simulink model "ACC_Main"  (R2026a)
settings: Solver=VariableStepAuto  StopTime=30
settings Model: Creator=Quang Huy  LastModifiedBy=ASUS

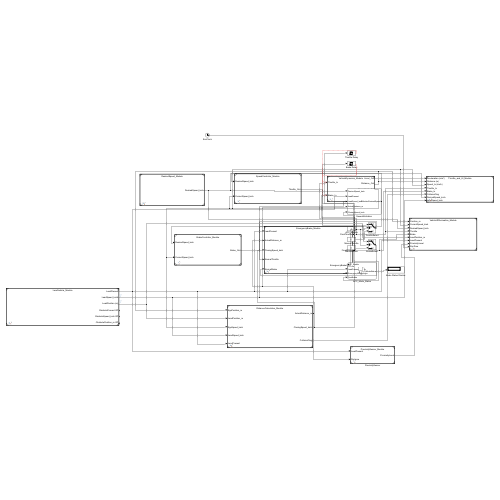
[thumbnail: Simulink's stored preview of the top-level diagram]
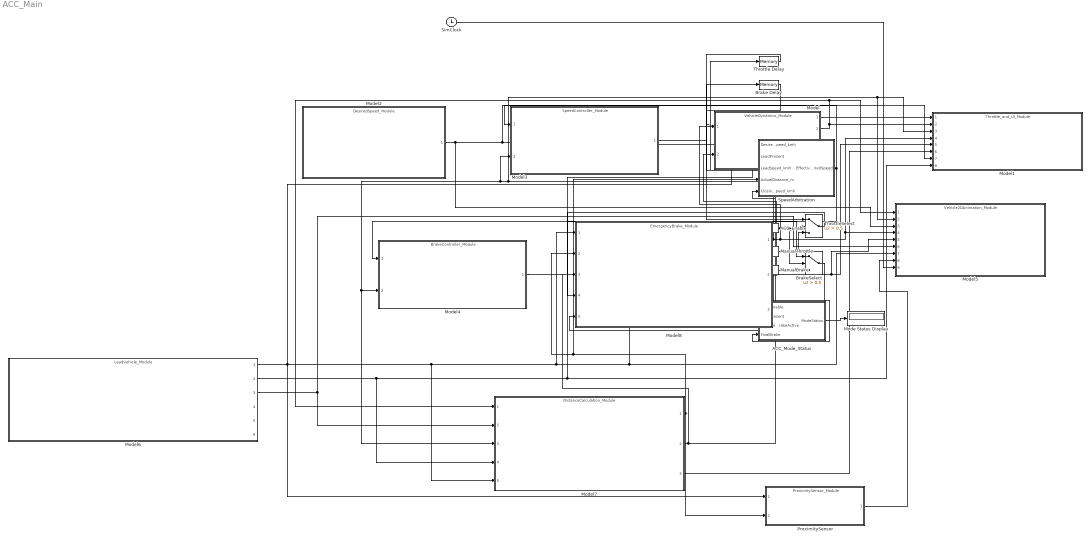
== system ACC_Main ==
  ACC_Enable : Constant  OutDataTypeStr=boolean
  ACC_Mode_Status : Stateflow chart  TreatAsAtomicUnit=on
  Brake Delay : Memory
  BrakeSelect : Switch  Criteria=u2 > Threshold  Threshold=0.5  SaturateOnIntegerOverflow=off  InputSameDT=off
  ManualBrake : Constant  Value=0
  ManualThrottle : Constant  Value=0  OutDataTypeStr=double
  Mode Status Display : Display
  Model : ModelReference  ModelNameDialog=VehicleDynamics_Module.slx  SimulationMode=Normal  ModelReferenceVersion=1.0
  Model1 : ModelReference  ModelNameDialog=Throttle_and_UI_Module.slx  SimulationMode=Normal  ModelReferenceVersion=3.2
  Model2 : ModelReference  ModelNameDialog=DesiredSpeed_Module.slx  SimulationMode=Normal  ModelReferenceVersion=1.0
  Model3 : ModelReference  ModelNameDialog=SpeedController_Module.slx  SimulationMode=Normal  ModelReferenceVersion=1.2
  Model4 : ModelReference  ModelNameDialog=BrakeController_Module.slx  SimulationMode=Normal  ModelReferenceVersion=1.0
  Model5 : ModelReference  ModelNameDialog=Vehicle2DAnimation_Module.slx  SimulationMode=Normal  ModelReferenceVersion=3.1
  Model6 : ModelReference  ModelNameDialog=LeadVehicle_Module.slx  SimulationMode=Normal  ModelReferenceVersion=3.1
  Model7 : ModelReference  ModelNameDialog=DistanceCalculation_Module.slx  SimulationMode=Normal  ModelReferenceVersion=1.0
  Model8 : ModelReference  ModelNameDialog=EmergencyBrake_Module.slx  SimulationMode=Normal  ModelReferenceVersion=1.0
  ProximitySensor : ModelReference  ModelNameDialog=ProximitySensor_Module.slx  SimulationMode=Normal  ModelReferenceVersion=1.2
  SimClock : Clock
  SpeedArbitration : Subsystem
  Throttle Delay : Memory
  ThrottleSelect : Switch  Criteria=u2 > Threshold  Threshold=0.5  SaturateOnIntegerOverflow=off  InputSameDT=off
  wires:
  Model2/1 -> SpeedArbitration/1(DesiredSpeed_kmh), Model1/7, Model5/3
  Model6/3 -> Model7/2, Model5/6
  Model6/2 -> SpeedArbitration/3(LeadSpeed_kmh), Model1/8, Model7/4
  Model8/1 -> Model1/4, Model5/4, Model/1, Throttle Delay/1
  Model8/2 -> Model1/5, Model5/5, Model/2, Brake Delay/1, ACC_Mode_Status/4(FinalBrake)
  Model7/2 -> Model8/3, SpeedArbitration/5(ClosingSpeed_kmh)
  Throttle Delay/1 -> ?
  Brake Delay/1 -> ?
  Model7/3 -> Model1/6
  SpeedArbitration/1(EffectiveDesiredSpeed) -> Model3/1, Model4/1
  Model3/1 -> ThrottleSelect/1
  ACC_Enable/1 -> ThrottleSelect/2, BrakeSelect/2, ACC_Mode_Status/1(ACC_Enable)
  ManualThrottle/1 -> ThrottleSelect/3
  ThrottleSelect/1 -> Model8/4
  Model4/1 -> BrakeSelect/1
  ManualBrake/1 -> BrakeSelect/3
  BrakeSelect/1 -> Model8/5
  Model8/3 -> ACC_Mode_Status/3(EmergencyBrakeActive)
  ACC_Mode_Status/1(ModeStatus) -> Mode Status Display/1
  Model6/1 -> Model5/7, ACC_Mode_Status/2(LeadPresent), Model8/1, Model7/5, ProximitySensor/1, SpeedArbitration/2(LeadPresent)
  Model7/1 -> Model8/2, SpeedArbitration/4(ActualDistance_m), ProximitySensor/2
  ProximitySensor/1 -> Model5/8
  SimClock/1 -> Model5/9
  Model/2 -> Model5/1, Model7/1, Model1/2
  Model/1 -> Model1/1
  Model/3 -> Model1/3, Model5/2, Model7/3, Model4/2, Model3/2

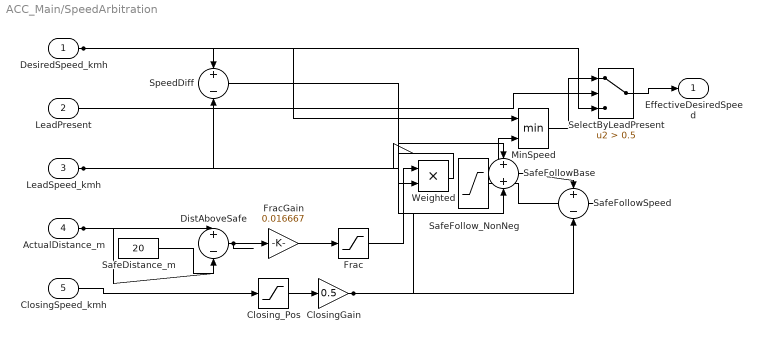
== system ACC_Main/SpeedArbitration ==
  DesiredSpeed_kmh : Inport
  LeadPresent : Inport  Port=2
  LeadSpeed_kmh : Inport  Port=3
  ActualDistance_m : Inport  Port=4
  ClosingSpeed_kmh : Inport  Port=5
  ClosingGain : Gain  Gain=0.5
  Closing_Pos : Saturate  UpperLimit=inf  LowerLimit=0
  DistAboveSafe : Sum  Inputs=+-
  Frac : Saturate  UpperLimit=1  LowerLimit=0
  FracGain : Gain  Gain=0.016667
  MinSpeed : MinMax  Inputs=2
  SafeDistance_m : Constant  Value=20
  SafeFollowBase : Sum
  SafeFollowSpeed : Sum  Inputs=+-
  SafeFollow_NonNeg : Saturate  UpperLimit=inf  LowerLimit=0
  SelectByLeadPresent : Switch  Criteria=u2 > Threshold  Threshold=0.5  SaturateOnIntegerOverflow=off  InputSameDT=off
  SpeedDiff : Sum  Inputs=+-
  Weighted : Product
  EffectiveDesiredSpeed : Outport
  wires:
  SafeDistance_m/1 -> DistAboveSafe/2
  ActualDistance_m/1 -> DistAboveSafe/1
  DistAboveSafe/1 -> FracGain/1
  ? -> ?
  ClosingSpeed_kmh/1 -> Closing_Pos/1
  Closing_Pos/1 -> ClosingGain/1
  LeadSpeed_kmh/1 -> SpeedDiff/2, SafeFollowBase/1
  ? -> ?
  ClosingGain/1 -> SafeFollowSpeed/2
  DesiredSpeed_kmh/1 -> MinSpeed/1, SelectByLeadPresent/3, SpeedDiff/1
  SafeFollow_NonNeg/1 -> MinSpeed/2
  MinSpeed/1 -> SelectByLeadPresent/1
  LeadPresent/1 -> SelectByLeadPresent/2
  SelectByLeadPresent/1 -> EffectiveDesiredSpeed/1
  FracGain/1 -> Frac/1
  Frac/1 -> Weighted/1
  SpeedDiff/1 -> Weighted/2
  Weighted/1 -> SafeFollowBase/2
  SafeFollowBase/1 -> SafeFollowSpeed/1
  SafeFollowSpeed/1 -> SafeFollow_NonNeg/1

== stateflow chart ACC_Main/ACC_Mode_Status ==
  state Off
    entry: ModeStatus = 0;
  state On
    during:
    if EmergencyBrakeActive
    ModeStatus = 4;
    elseif FinalBrake > 0
    ModeStatus = 3;
    elseif LeadPresent
    ModeStatus = 2;
    else
    ModeStatus = 1;
    end
  On -> Off : [~ACC_Enable]
  (default) -> Off
  Off -> On : [ACC_Enable]
  data: ACC_Enable input boolean; LeadPresent input boolean; EmergencyBrakeActive input boolean; FinalBrake input double; ModeStatus output uint8
